simulink model "chap2_1sim"  (R2015a)
settings: Solver=ode45  StartTime=0.0  StopTime=RunTime  RelTol=1e-3
settings Model: Creator=Masoud  LastModifiedBy=MSD
settings DebuggingCC: InheritedTsInSrcMsg=none  DiscreteInheritContinuousMsg=none

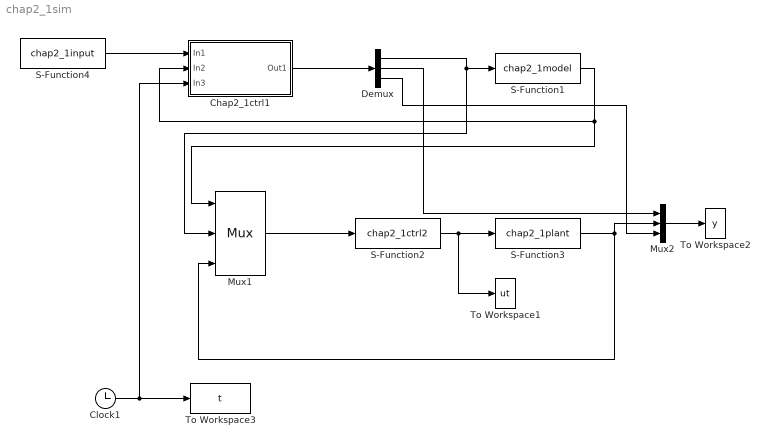
== system chap2_1sim ==
  Chap2_1ctrl1 : Subsystem
  Clock1 : Clock
  Demux : Demux  Outputs=3
  Mux1 : Mux  Inputs=3
  Mux2 : Mux  Inputs=3
  S-Function1 : S-Function  FunctionName=chap2_1model  SFunctionModules='chap2_1model'
  S-Function2 : S-Function  FunctionName=chap2_1ctrl2  SFunctionModules='chap2_1ctrl2'
  S-Function3 : S-Function  FunctionName=chap2_1plant  SFunctionModules='chap2_1plant'
  S-Function4 : S-Function  FunctionName=chap2_1input  SFunctionModules='chap2_1input'
  To Workspace1 : ToWorkspace  VariableName=ut  SampleTime=-1
  To Workspace2 : ToWorkspace  VariableName=y  SampleTime=-1
  To Workspace3 : ToWorkspace  VariableName=t  SampleTime=-1
  wires:
  S-Function1/1 -> Mux1/1, Chap2_1ctrl1/2(In2)
  S-Function2/1 -> To Workspace1/1, S-Function3/1
  Mux1/1 -> S-Function2/1
  S-Function3/1 -> Mux2/2, Mux1/3
  Mux2/1 -> To Workspace2/1
  Demux/1 -> S-Function1/1, Mux1/2
  Demux/2 -> Mux2/1
  Demux/3 -> Mux2/3
  Clock1/1 -> To Workspace3/1, Chap2_1ctrl1/3(In3)
  S-Function4/1 -> Chap2_1ctrl1/1(In1)
  Chap2_1ctrl1/1(Out1) -> Demux/1

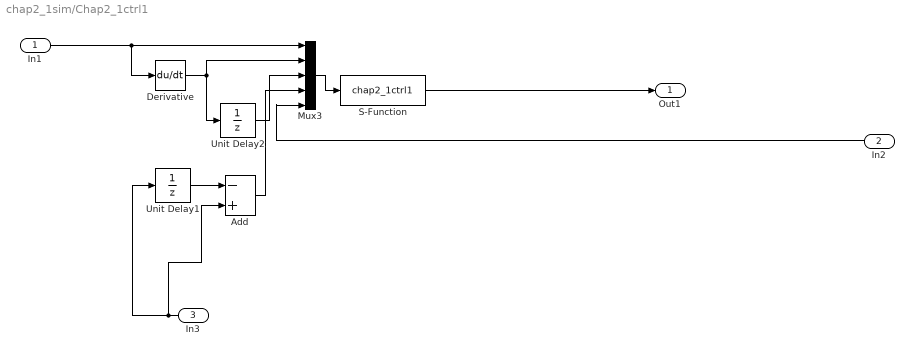
== system chap2_1sim/Chap2_1ctrl1 ==
  In1 : Inport
  In2 : Inport  Port=2
  In3 : Inport  Port=3
  Add : Sum  Inputs=-+
  Derivative : Derivative
  Mux3 : Mux  Inputs=5
  S-Function : S-Function  FunctionName=chap2_1ctrl1  SFunctionModules='chap2_1ctrl1'
  Unit Delay1 : UnitDelay  SampleTime=-1
  Unit Delay2 : UnitDelay  SampleTime=-1
  Out1 : Outport
  wires:
  S-Function/1 -> Out1/1
  In3/1 -> Add/2, Unit Delay1/1
  In2/1 -> Mux3/5
  Unit Delay2/1 -> Mux3/3
  Derivative/1 -> Mux3/2, Unit Delay2/1
  Mux3/1 -> S-Function/1
  Add/1 -> Mux3/4
  In1/1 -> Derivative/1, Mux3/1
  Unit Delay1/1 -> Add/1
